simulink model "simulation_loop"  (R2014a)
settings: Solver=ode45  StartTime=0.0  StopTime=20  RelTol=1e-3
settings Model: Creator=kadir  LastModifiedBy=kadir

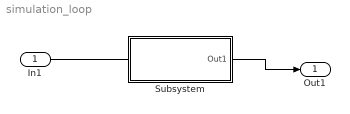
== system simulation_loop ==
  In1 : Inport
  Subsystem : Subsystem
  Out1 : Outport
  wires:
  Subsystem/1(Out1) -> Out1/1
  In1/1 -> ?

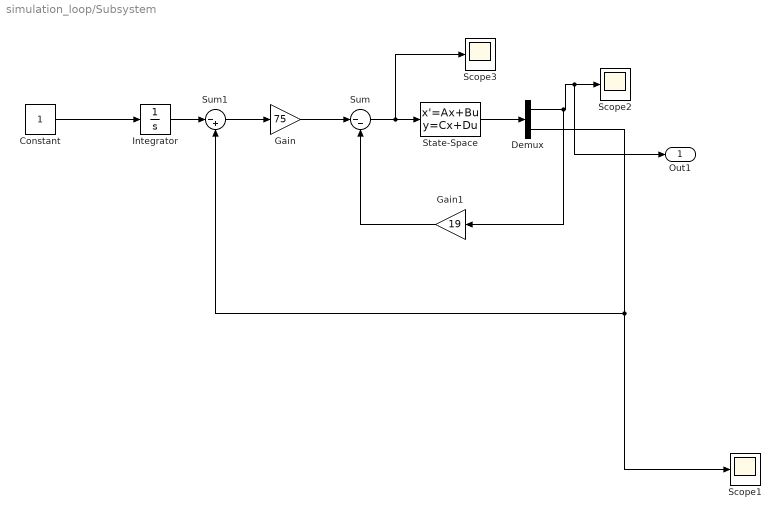
== system simulation_loop/Subsystem ==
  Constant : Constant
  Demux : Demux  Outputs=2
  Gain : Gain  Gain=75
  Gain1 : Gain  Gain=19
  Integrator : Integrator
  Scope1 : Scope
  Scope2 : Scope
      settings: SaveName=ScopeData2
  Scope3 : Scope
  State-Space : StateSpace  A=[-0.1333 0;1 0]  B=[0.6667 0]'  C=[1 0; 0 1]  D=[0 0]'  X0=[0 0]
  Sum : Sum  Inputs=|--
  Sum1 : Sum  Inputs=|-+
  Out1 : Outport
  wires:
  Sum/1 -> Scope3/1, State-Space/1
  Gain/1 -> Sum/1
  State-Space/1 -> Demux/1
  Demux/1 -> Gain1/1, Out1/1, Scope2/1
  Gain1/1 -> Sum/2
  Integrator/1 -> Sum1/1
  Sum1/1 -> Gain/1
  Demux/2 -> Sum1/2, Scope1/1
  Constant/1 -> Integrator/1
